simulink model "MOIsolatedBuck2"  (R2013a)
settings: Solver=ode45  StartTime=0.0  StopTime=0.25  RelTol=1e-3
libraries: powerlib x43
settings Model: Creator=Sony  LastModifiedBy=Sony

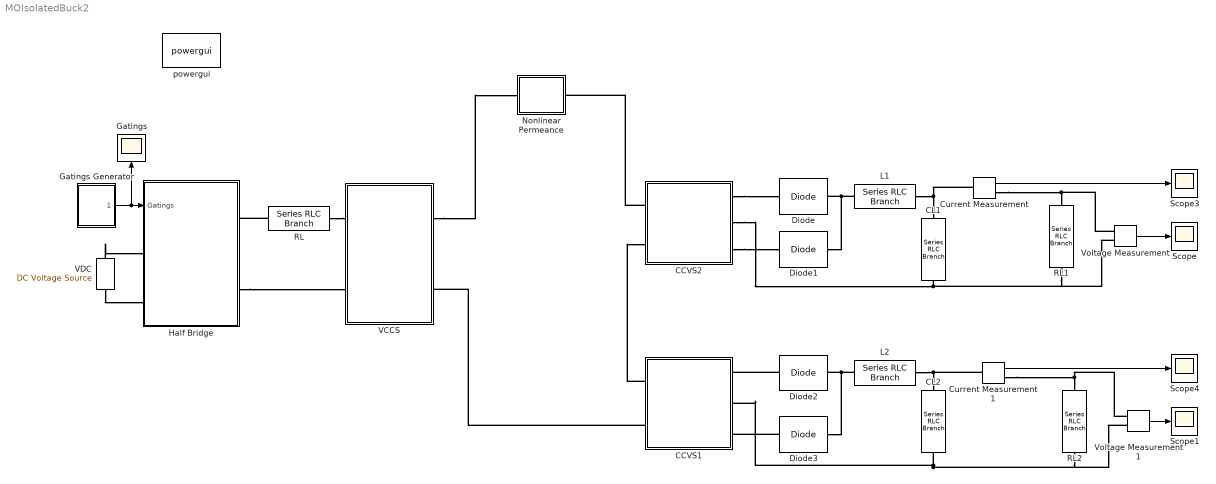
== system MOIsolatedBuck2 ==
  CCVS1 : Subsystem  mask{N=30}
  CCVS2 : Subsystem  mask{N=10}
  CL1 : powerlib/Elements/Series RLC Branch  LConnTagsString=__new0  RConnTagsString=__new0  BranchType=C  Resistance=1  Inductance=1e-3  SetiL0=off  InitialCurrent=0  Capacitance=1e-5  Setx0=off  InitialVoltage=0  Measurements=None
  CL2 : powerlib/Elements/Series RLC Branch  LConnTagsString=__new0  RConnTagsString=__new0  BranchType=C  Resistance=1  Inductance=1e-3  SetiL0=off  InitialCurrent=0  Capacitance=1e-5  Setx0=off  InitialVoltage=0  Measurements=None
  Current Measurement : powerlib/Measurements/Current Measurement  PhasorSimulation=off  OutputType=Complex  PSBequivalent=0
  Current Measurement1 : powerlib/Measurements/Current Measurement  PhasorSimulation=off  OutputType=Complex  PSBequivalent=0
  Diode{,1..3} (4 alike) : powerlib/Power Electronics/Diode  Ron=1e-3  Lon=0  Vf=0  IC=0  UseSnubber=off  Rs=500  Cs=250e-9  Measurements=off
  Gatings : Scope
      settings: YMin=0  YMax=608000  SaveName=ScopeData2
  Gatings Generator : Subsystem  mask{Fs=75000, D=75}
  Half Bridge : Subsystem
  L1 : powerlib/Elements/Series RLC Branch  LConnTagsString=__new0  RConnTagsString=__new0  BranchType=L  Resistance=1  Inductance=1e-3  SetiL0=off  InitialCurrent=0  Capacitance=1e-6  Setx0=off  InitialVoltage=0  Measurements=None
  L2 : powerlib/Elements/Series RLC Branch  LConnTagsString=__new0  RConnTagsString=__new0  BranchType=L  Resistance=1  Inductance=1e-3  SetiL0=off  InitialCurrent=0  Capacitance=1e-6  Setx0=off  InitialVoltage=0  Measurements=None
  Nonlinear Permeance : Subsystem  mask{R=1e9, C=1.7e-5}
  RL : powerlib/Elements/Series RLC Branch  LConnTagsString=__new0  RConnTagsString=__new0  BranchType=RL  Resistance=1  Inductance=1e-5  SetiL0=off  InitialCurrent=0  Capacitance=1e-6  Setx0=off  InitialVoltage=0  Measurements=None
  RL1 : powerlib/Elements/Series RLC Branch  LConnTagsString=__new0  RConnTagsString=__new0  BranchType=R  Resistance=1/20  Inductance=1e-3  SetiL0=off  InitialCurrent=0  Capacitance=1e-6  Setx0=off  InitialVoltage=0  Measurements=None
  RL2 : powerlib/Elements/Series RLC Branch  LConnTagsString=__new0  RConnTagsString=__new0  BranchType=R  Resistance=1  Inductance=1e-3  SetiL0=off  InitialCurrent=0  Capacitance=1e-6  Setx0=off  InitialVoltage=0  Measurements=None
  Scope{,1,3..4} (4 alike) : Scope
      Scope settings: YMin=0  YMax=10  SaveName=Vou
      Scope1 settings: YMin=0  YMax=17.245  SaveName=Vol
      Scope3 settings: YMin=0  YMax=150  SaveName=Iou
      Scope4 settings: YMin=10  YMax=20.5  SaveName=Iol
  VCCS : Subsystem  mask{N=110}
  VDC : powerlib/Electrical Sources/DC Voltage Source  Amplitude=160  Measurements=None
  Voltage Measurement : powerlib/Measurements/Voltage Measurement  PhasorSimulation=off  OutputType=Complex  PSBequivalent=0
  Voltage Measurement1 : powerlib/Measurements/Voltage Measurement  PhasorSimulation=off  OutputType=Complex  PSBequivalent=0
  powergui : powerlib/powergui  Priority=1  SimulationMode=Continuous  SolverType=Backward Euler  SampleTime=1e-5  frequency=60  SPID=on  DisableSnubberDevices=off  DisableRonSwitches=off  DisableVfSwitches=off  SwTol=0  Interpol=off  DisplayEquations=off  frequencyindice=0  Pbase=100e6  ErrMax=1e-4  Iterations=50  UnitsV=kV  UnitsW=MW  FunctionMessages=off  echomessages=off  HookPort=off  EnableUseOfTLC=off  x0status=blocks  RestoreLinks=warning  ResistiveCurrentMeasurement=off  Frange=[0:2:500]  Ylog=off  Xlog=on  ShowGrid=off  save=off  variable=ZData  ZoomFFT=off  StartTime=0.0  cycles=1  DisplayStyle=1  fundamental=60  FreqAxis=off  MaxFrequency=1000  frequencyindicesteady=1  RmsSteady=1  display=off  Ts=0  methode=off
  wires:
  Gatings Generator/1(Gatings) -> Gatings/1, Half Bridge/1(Gatings)
  Voltage Measurement/1 -> Scope/1
  Voltage Measurement1/1 -> Scope1/1
  Current Measurement/1 -> Scope3/1
  Current Measurement1/1 -> Scope4/1
  connections:
  VDC/RConn1 -- Half Bridge/LConn1
  VDC/LConn1 -- Half Bridge/LConn2
  RL/LConn1 -- Half Bridge/RConn1
  Half Bridge/RConn2 -- VCCS/LConn2
  CCVS2/RConn1 -- Diode/LConn1
  CCVS2/RConn3 -- Diode1/LConn1
  CCVS2/RConn2 -- Voltage Measurement/LConn2 -- RL1/LConn1 -- CL1/LConn1
  CL2/LConn1 -- CCVS1/RConn2 -- Voltage Measurement1/LConn2 -- RL2/LConn1
  Diode3/RConn1 -- L2/RConn1 -- Diode2/RConn1
  Diode3/LConn1 -- CCVS1/RConn3
  Diode2/LConn1 -- CCVS1/RConn1
  VCCS/RConn1 -- Nonlinear Permeance/LConn1
  Diode1/RConn1 -- L1/RConn1 -- Diode/RConn1
  Voltage Measurement1/LConn1 -- Current Measurement1/RConn1 -- RL2/RConn1
  L1/LConn1 -- CL1/RConn1 -- Current Measurement/LConn1
  L2/LConn1 -- Current Measurement1/LConn1 -- CL2/RConn1
  Voltage Measurement/LConn1 -- Current Measurement/RConn1 -- RL1/RConn1
  CCVS1/LConn1 -- CCVS2/LConn2
  RL/RConn1 -- VCCS/LConn1
  CCVS2/LConn1 -- Nonlinear Permeance/RConn1
  CCVS1/LConn2 -- VCCS/RConn2

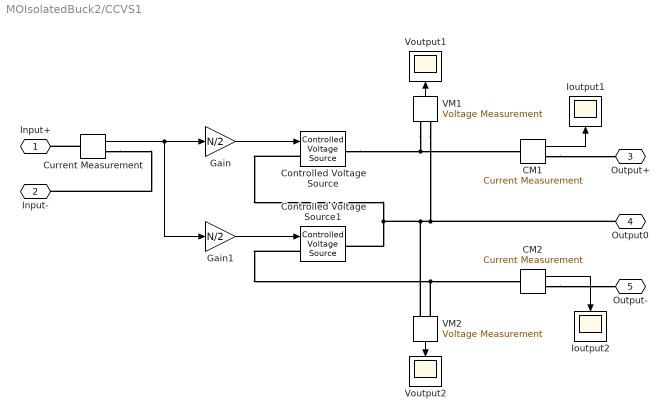
== system MOIsolatedBuck2/CCVS1 ==
  CM1 : powerlib/Measurements/Current Measurement  PhasorSimulation=off  OutputType=Complex  PSBequivalent=0
  CM2 : powerlib/Measurements/Current Measurement  PhasorSimulation=off  OutputType=Complex  PSBequivalent=0
  Controlled Voltage Source : powerlib/Electrical Sources/Controlled Voltage Source  Initialize=on  Source_Type=AC  Amplitude=0  Phase=0  Frequency=0  Measurements=None
  Controlled Voltage Source1 : powerlib/Electrical Sources/Controlled Voltage Source  Initialize=on  Source_Type=AC  Amplitude=0  Phase=0  Frequency=0  Measurements=None
  Current Measurement : powerlib/Measurements/Current Measurement  PhasorSimulation=off  OutputType=Complex  PSBequivalent=0
  Gain : Gain  Gain=N/2
  Gain1 : Gain  Gain=N/2
  Ioutput1 : Scope
      settings: YMin=-25  YMax=150  SaveName=Iolp
  Ioutput2 : Scope
      settings: YMin=-10  YMax=150  SaveName=Ioln
  VM1 : powerlib/Measurements/Voltage Measurement  PhasorSimulation=off  OutputType=Complex  PSBequivalent=0
  VM2 : powerlib/Measurements/Voltage Measurement  PhasorSimulation=off  OutputType=Complex  PSBequivalent=0
  Voutput1 : Scope
      settings: YMin=-100  YMax=100  SaveName=Volp
  Voutput2 : Scope
      settings: YMin=-175  YMax=175  SaveName=Voln
  Input+ : PMIOPort  Port=1  Side=Left
  Input- : PMIOPort  Port=2  Side=Left
  Output+ : PMIOPort  Port=3  Side=Right
  Output0 : PMIOPort  Port=4  Side=Right
  Output- : PMIOPort  Port=5  Side=Right
  wires:
  Gain/1 -> Controlled Voltage Source/1
  Current Measurement/1 -> Gain1/1, Gain/1
  Gain1/1 -> Controlled Voltage Source1/1
  VM2/1 -> Voutput2/1
  VM1/1 -> Voutput1/1
  CM2/1 -> Ioutput2/1
  CM1/1 -> Ioutput1/1
  connections:
  Current Measurement/LConn1 -- Input+/RConn1
  Current Measurement/RConn1 -- Input-/RConn1
  VM1/LConn1 -- Controlled Voltage Source/RConn1 -- CM1/LConn1
  Output0/RConn1 -- VM2/LConn1 -- Controlled Voltage Source1/RConn1 -- Controlled Voltage Source/LConn1 -- VM1/LConn2
  VM2/LConn2 -- Controlled Voltage Source1/LConn1 -- CM2/LConn1
  CM1/RConn1 -- Output+/RConn1
  CM2/RConn1 -- Output-/RConn1

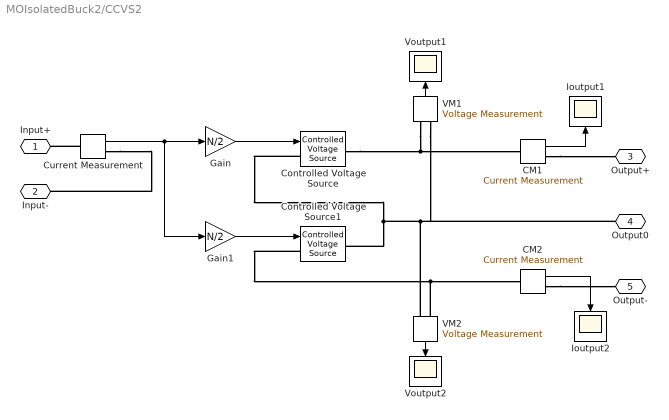
== system MOIsolatedBuck2/CCVS2 ==
  CM1 : powerlib/Measurements/Current Measurement  PhasorSimulation=off  OutputType=Complex  PSBequivalent=0
  CM2 : powerlib/Measurements/Current Measurement  PhasorSimulation=off  OutputType=Complex  PSBequivalent=0
  Controlled Voltage Source : powerlib/Electrical Sources/Controlled Voltage Source  Initialize=on  Source_Type=AC  Amplitude=0  Phase=0  Frequency=0  Measurements=None
  Controlled Voltage Source1 : powerlib/Electrical Sources/Controlled Voltage Source  Initialize=on  Source_Type=AC  Amplitude=0  Phase=0  Frequency=0  Measurements=None
  Current Measurement : powerlib/Measurements/Current Measurement  PhasorSimulation=off  OutputType=Complex  PSBequivalent=0
  Gain : Gain  Gain=N/2
  Gain1 : Gain  Gain=N/2
  Ioutput1 : Scope
      settings: YMin=-25  YMax=150  SaveName=Ioup
  Ioutput2 : Scope
      settings: YMin=-10  YMax=150  SaveName=Ioun
  VM1 : powerlib/Measurements/Voltage Measurement  PhasorSimulation=off  OutputType=Complex  PSBequivalent=0
  VM2 : powerlib/Measurements/Voltage Measurement  PhasorSimulation=off  OutputType=Complex  PSBequivalent=0
  Voutput1 : Scope
      settings: YMin=-20  YMax=20  SaveName=Voup
  Voutput2 : Scope
      settings: YMin=-20  YMax=20  SaveName=Voun
  Input+ : PMIOPort  Port=1  Side=Left
  Input- : PMIOPort  Port=2  Side=Left
  Output+ : PMIOPort  Port=3  Side=Right
  Output0 : PMIOPort  Port=4  Side=Right
  Output- : PMIOPort  Port=5  Side=Right
  wires:
  Gain/1 -> Controlled Voltage Source/1
  Current Measurement/1 -> Gain1/1, Gain/1
  Gain1/1 -> Controlled Voltage Source1/1
  VM2/1 -> Voutput2/1
  VM1/1 -> Voutput1/1
  CM2/1 -> Ioutput2/1
  CM1/1 -> Ioutput1/1
  connections:
  Current Measurement/LConn1 -- Input+/RConn1
  Current Measurement/RConn1 -- Input-/RConn1
  Controlled Voltage Source/RConn1 -- CM1/LConn1 -- VM1/LConn1
  Controlled Voltage Source/LConn1 -- Output0/RConn1 -- VM1/LConn2 -- VM2/LConn1 -- Controlled Voltage Source1/RConn1
  Controlled Voltage Source1/LConn1 -- VM2/LConn2 -- CM2/LConn1
  CM1/RConn1 -- Output+/RConn1
  CM2/RConn1 -- Output-/RConn1

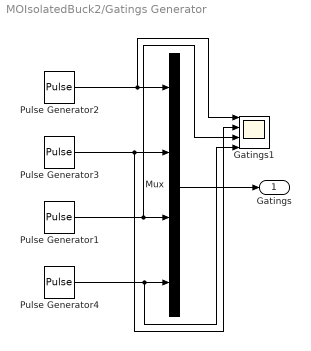
== system MOIsolatedBuck2/Gatings Generator ==
  Gatings1 : Scope  NumInputPorts=4
      settings: YMin=-1~-1~-1~-1  YMax=2~2~2~2  SaveName=ScopeData3
  Mux : Mux
  Pulse Generator1 : DiscretePulseGenerator  PulseType=Time based  Period=1/Fs  PulseWidth=100-D  PhaseDelay=(D)/(100*Fs)
  Pulse Generator2 : DiscretePulseGenerator  PulseType=Time based  Period=1/Fs  PulseWidth=D
  Pulse Generator3 : DiscretePulseGenerator  PulseType=Time based  Period=1/Fs  PulseWidth=100-D  PhaseDelay=(D)/(100*Fs)
  Pulse Generator4 : DiscretePulseGenerator  PulseType=Time based  Period=1/Fs  PulseWidth=D
  Gatings : Outport
  wires:
  Mux/1 -> Gatings/1
  Pulse Generator2/1 -> Gatings1/1, Mux/1
  Pulse Generator1/1 -> Gatings1/3, Mux/3
  Pulse Generator3/1 -> Gatings1/2, Mux/2
  Pulse Generator4/1 -> Gatings1/4, Mux/4

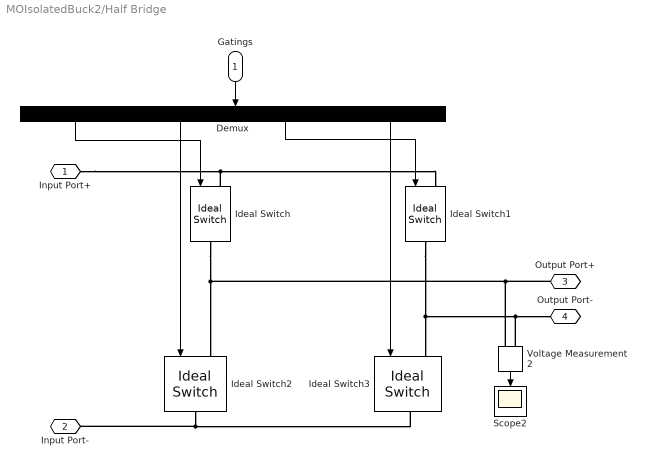
== system MOIsolatedBuck2/Half Bridge ==
  Gatings : Inport
  Demux : Demux
  Ideal Switch{,1..3} (4 alike) : powerlib/Power Electronics/Ideal Switch  Ron=0.001  Lon=0  IC=0  Rs=1e5  Cs=inf  Measurements=off
  Scope2 : Scope
      settings: YMin=-175  YMax=175  SaveName=Vinput
  Voltage Measurement2 : powerlib/Measurements/Voltage Measurement  PhasorSimulation=off  OutputType=Complex  PSBequivalent=0
  Input Port+ : PMIOPort  Port=1  Side=Left
  Input Port- : PMIOPort  Port=2  Side=Left
  Output Port+ : PMIOPort  Port=3  Side=Right
  Output Port- : PMIOPort  Port=4  Side=Right
  wires:
  Demux/3 -> Ideal Switch1/1
  Demux/1 -> Ideal Switch/1
  Demux/2 -> Ideal Switch2/1
  Gatings/1 -> Demux/1
  Demux/4 -> Ideal Switch3/1
  Voltage Measurement2/1 -> Scope2/1
  connections:
  Ideal Switch/LConn1 -- Ideal Switch1/LConn1 -- Input Port+/RConn1
  Ideal Switch2/RConn1 -- Ideal Switch3/RConn1 -- Input Port-/RConn1
  Ideal Switch1/RConn1 -- Ideal Switch3/LConn1 -- Voltage Measurement2/LConn2 -- Output Port-/RConn1
  Ideal Switch/RConn1 -- Voltage Measurement2/LConn1 -- Output Port+/RConn1 -- Ideal Switch2/LConn1

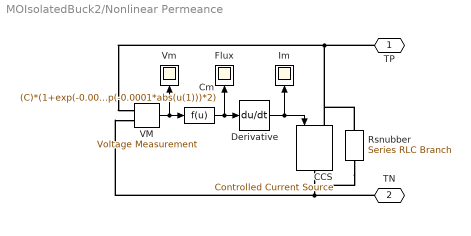
== system MOIsolatedBuck2/Nonlinear Permeance ==
  CCS : powerlib/Electrical Sources/Controlled Current Source  Initialize=on  Source_Type=AC  Amplitude=0  Phase=0  Frequency=0  Measurements=None
  Cm : Fcn  Expr=(C)*(1+exp(-0.0001*abs(u(1)))*1-exp(-0.0001*abs(u(1)))*2)
  Derivative : Derivative
  Flux : Scope
      settings: YMin=5.5e-06  YMax=1.25e-05  SaveName=PermeanceFlux
  Im : Scope
      settings: TimeRange=0.12  YMin=-0.0001  YMax=0.0001  SaveName=PermeanceIm
  Rsnubber : powerlib/Elements/Series RLC Branch  LConnTagsString=__new0  RConnTagsString=__new0  BranchType=R  Resistance=R  Inductance=1e-3  SetiL0=off  InitialCurrent=0  Capacitance=1e-6  Setx0=off  InitialVoltage=0  Measurements=None
  VM : powerlib/Measurements/Voltage Measurement  PhasorSimulation=off  OutputType=Complex  PSBequivalent=0
  Vm : Scope
      settings: YMin=-13000  YMax=-4000  SaveName=PermeanceVm
  TP : PMIOPort  Port=1  Side=Left
  TN : PMIOPort  Port=2  Side=Right
  wires:
  VM/1 -> Vm/1, Cm/1
  Cm/1 -> Flux/1, Derivative/1
  Derivative/1 -> Im/1, CCS/1
  connections:
  TN/RConn1 -- Rsnubber/RConn1 -- CCS/RConn1 -- VM/LConn2
  TP/RConn1 -- Rsnubber/LConn1 -- CCS/LConn1 -- VM/LConn1

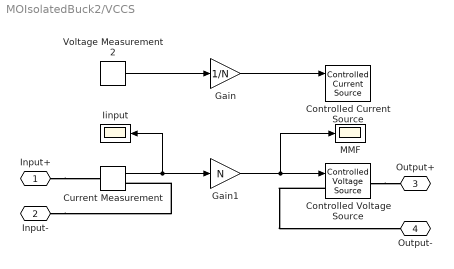
== system MOIsolatedBuck2/VCCS ==
  Controlled Current Source : powerlib/Electrical Sources/Controlled Current Source  Initialize=on  Source_Type=AC  Amplitude=0  Phase=0  Frequency=0  Measurements=None
  Controlled Voltage Source : powerlib/Electrical Sources/Controlled Voltage Source  Initialize=off  Source_Type=AC  Amplitude=0  Phase=0  Frequency=0  Measurements=None
  Current Measurement : powerlib/Measurements/Current Measurement  PhasorSimulation=off  OutputType=Complex  PSBequivalent=0
  Gain : Gain  Gain=1/N
  Gain1 : Gain  Gain=N
  Iinput : Scope
      settings: YMin=0  YMax=150  SaveName=Iprimary
  MMF : Scope
      settings: YMin=0  YMax=15000  SaveName=MMF
  Voltage Measurement2 : powerlib/Measurements/Voltage Measurement  PhasorSimulation=off  OutputType=Complex  PSBequivalent=0
  Input+ : PMIOPort  Port=1  Side=Left
  Input- : PMIOPort  Port=2  Side=Left
  Output+ : PMIOPort  Port=3  Side=Right
  Output- : PMIOPort  Port=4  Side=Right
  wires:
  Gain/1 -> Controlled Current Source/1
  Voltage Measurement2/1 -> Gain/1
  Current Measurement/1 -> Iinput/1, Gain1/1
  Gain1/1 -> MMF/1, Controlled Voltage Source/1
  connections:
  Input+/RConn1 -- Current Measurement/LConn1
  Input-/RConn1 -- Current Measurement/RConn1
  Controlled Voltage Source/RConn1 -- Output+/RConn1
  Controlled Voltage Source/LConn1 -- Output-/RConn1
